simulink model "simulator_model_PVA_FINAL"  (R2016b)
settings: Solver=FixedStepAuto  StartTime=0.0  StopTime=t  FixedStep=0.005  RelTol=1e-3
StopFcn:
  | Plots
values from neighbouring files (symbols this model uses):
  a_cross = exp(-deltat/tau)    [simulation_script.m]
  a_long = a_cross    [simulation_script.m]
  a_vel_att = exp(-deltat/tau_vel_att)    [simulation_script.m]
  deltat = deltat_array(i)    [simulation_script.m]
  lat = latency(h)*0.001    [simulation_script.m]
  lat_acc = 3.25    [simulation_script.m]
  s_att = sqrt(1-a_vel_att^2)*s_att_e    [simulation_script.m]
  s_cross = sqrt(1-a_cross^2)*s_e(k)    [simulation_script.m]
  s_long = sqrt(1-a_long^2)*s_e1(k)    [simulation_script.m]
  s_vel = sqrt(1-a_vel_att^2)*s_vel_e    [simulation_script.m]
libraries: simulink x3
settings Model: Creator=trrrbe  LastModifiedBy=trrrbe
settings SolverCC: ZeroCrossAlgorithm=Adaptive
settings OptimizationCC: EfficientFloat2IntCast=on

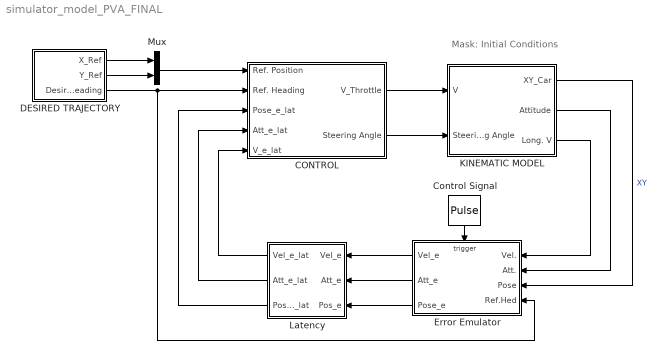
== system simulator_model_PVA_FINAL ==
  note: Mask: Initial Conditions
  CONTROL : Subsystem
  Control Signal : DiscretePulseGenerator  PulseType=Time based  Period=deltat  PulseWidth=50
  DESIRED TRAJECTORY : Subsystem  mask{n=3, A=100}
      mask prompts: n "Eccentricity"; A "Amplitude"
  Error Emulator : Subsystem
  KINEMATIC MODEL : Subsystem  mask{ref=0, x0=0, y0=0}
      mask prompts: ref "Reference Heading"; x0 "Initial Position X"; y0 "Initial Position Y"
  Latency : Subsystem
  Mux : Mux  Inputs=2
  wires:
  KINEMATIC MODEL/1(XY_Car) -> Error Emulator/3(Pose)  "XY"
  CONTROL/1(V_Throttle) -> KINEMATIC MODEL/1(V)
  DESIRED TRAJECTORY/1(X_Ref) -> Mux/1
  DESIRED TRAJECTORY/2(Y_Ref) -> Mux/2
  KINEMATIC MODEL/3(Long. V) -> Error Emulator/1(Vel.)
  KINEMATIC MODEL/2(Attitude) -> Error Emulator/2(Att.)
  DESIRED TRAJECTORY/3(Desired Heading) -> Error Emulator/4("Ref.Hed "), CONTROL/2(Ref. Heading)
  Control Signal/1 -> Error Emulator/Trigger
  Error Emulator/1(Vel_e) -> Latency/1(Vel_e)
  Error Emulator/3(Pose_e) -> Latency/3(Pos_e)
  CONTROL/2(Steering Angle) -> KINEMATIC MODEL/2(Steering Angle)
  Latency/3(Pos_e_lat) -> CONTROL/3(Pose_e_lat)
  Latency/1(Vel_e_lat) -> CONTROL/5(V_e_lat)
  Latency/2(Att_e_lat) -> CONTROL/4(Att_e_lat)
  Mux/1 -> CONTROL/1(Ref. Position)
  Error Emulator/2(Att_e) -> Latency/2(Att_e)

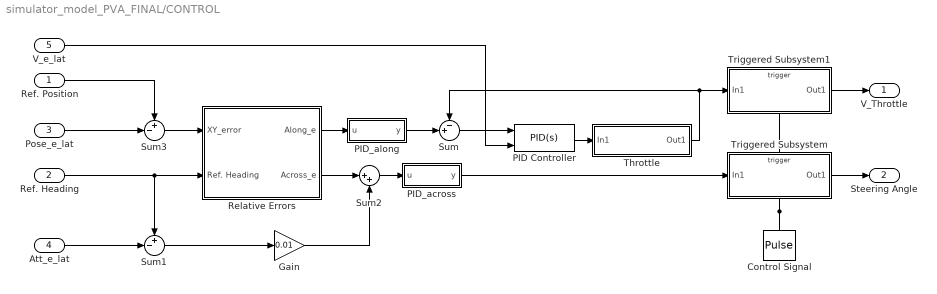
== system simulator_model_PVA_FINAL/CONTROL ==
  Ref. Position : Inport
  Ref. Heading : Inport  Port=2
  Pose_e_lat : Inport  Port=3
  Att_e_lat : Inport  Port=4
  V_e_lat : Inport  Port=5
  Control Signal : DiscretePulseGenerator  PulseType=Time based  Period=deltat  PulseWidth=50
  Gain : Gain  Gain=0.01
  PID Controller : simulink/Continuous/PID Controller  Controller=PID  TimeDomain=Continuous-time  SampleTime=-1  IntegratorMethod=Forward Euler  FilterMethod=Forward Euler  Form=Parallel  UseFilter=on  ControllerParametersSource=internal  P=209.609082036899  I=13.2325958582808  D=596.721506223276  N=1.87779602070702  InitialConditionSource=internal  InitialConditionForIntegrator=0  InitialConditionForFilter=0  ExternalReset=none  LimitOutput=off  UpperSaturationLimit=inf  LowerSaturationLimit=0  LinearizeAsGain=off  AntiWindupMode=clamping  Kb=1000  TrackingMode=on  Kt=t/500  PParamMin=[]  PParamMax=[]  IParamMin=[]  IParamMax=[]  DParamMin=[]  DParamMax=[]  NParamMin=[]  NParamMax=[]  KbParamMin=[]  KbParamMax=[]  KtParamMin=[]  KtParamMax=[]  POutMin=[]  POutMax=[]  IOutMin=[]  IOutMax=[]  DOutMin=[]  DOutMax=[]  NOutMin=[]  NOutMax=[]  KbOutMin=[]  KbOutMax=[]  KtOutMin=[]  KtOutMax=[]  IntegratorOutMin=[]  IntegratorOutMax=[]  FilterOutMin=[]  FilterOutMax=[]  SumOutMin=[]  SumOutMax=[]  SumI1OutMin=[]  SumI1OutMax=[]  SumI2OutMin=[]  SumI2OutMax=[]  SumI3OutMin=[]  SumI3OutMax=[]  SumDOutMin=[]  SumDOutMax=[]  SaturationOutMin=[]  SaturationOutMax=[]  IntegratorContinuousStateAttributes=''  IntegratorStateMustResolveToSignalObject=off  IntegratorRTWStateStorageClass=Auto  FilterContinuousStateAttributes=''  FilterStateMustResolveToSignalObject=off  FilterRTWStateStorageClass=Auto  DifferentiatorICPrevScaledInput=0  DifferentiatorOutMin=[]  DifferentiatorOutMax=[]
  PID_across : Subsystem
  PID_along : Subsystem
  Relative Errors : Subsystem
  Sum : Sum  Inputs=-+|
  Sum1 : Sum  Inputs=+-|
  Sum2 : Sum  Inputs=|++
  Sum3 : Sum  Inputs=+-|
  Throttle : Subsystem
  Triggered Subsystem : Subsystem  TreatAsAtomicUnit=on
  Triggered Subsystem1 : Subsystem  TreatAsAtomicUnit=on
  V_Throttle : Outport
  Steering Angle : Outport  Port=2
  wires:
  PID Controller/1 -> Throttle/1(In1)
  Sum/1 -> PID Controller/1
  Pose_e_lat/1 -> Sum3/2
  Ref. Position/1 -> Sum3/1
  Ref. Heading/1 -> Relative Errors/2(Ref. Heading), Sum1/1
  Att_e_lat/1 -> Sum1/2
  Throttle/1(Out1) -> Triggered Subsystem1/1(In1), Sum/1
  Triggered Subsystem/1(Out1) -> Steering Angle/1
  Control Signal/1 -> Triggered Subsystem/Trigger, Triggered Subsystem1/Trigger
  Sum3/1 -> Relative Errors/1(XY_error)
  Triggered Subsystem1/1(Out1) -> V_Throttle/1
  Relative Errors/1(Along_e) -> PID_along/1(u)
  Relative Errors/2(Across_e) -> Sum2/1
  PID_along/1(y) -> Sum/2
  Sum1/1 -> Gain/1
  V_e_lat/1 -> PID Controller/2
  Sum2/1 -> PID_across/1(u)
  PID_across/1(y) -> Triggered Subsystem/1(In1)
  Gain/1 -> Sum2/2

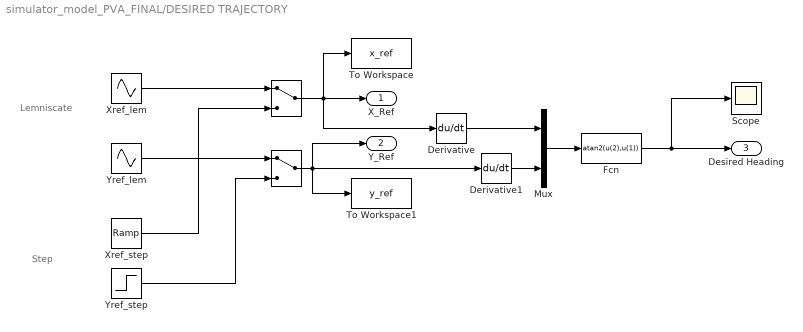
== system simulator_model_PVA_FINAL/DESIRED TRAJECTORY ==
  note: Step
  note: Lemniscate
  " " : ManualSwitch
  "  " : ManualSwitch
  Derivative : Derivative
  Derivative1 : Derivative
  Fcn : Fcn  Expr=atan2(u(2),u(1))
  Mux : Mux  Inputs=2
  Scope : Scope
  To Workspace : ToWorkspace  VariableName=x_ref  SaveFormat=Timeseries  SampleTime=-1
  To Workspace1 : ToWorkspace  VariableName=y_ref  SaveFormat=Timeseries  SampleTime=-1
  Xref_lem : Sin  Amplitude=n*A  Frequency=2*pi/t  SampleTime=0
  Xref_step : simulink/Sources/Ramp  slope=10  start=0  X0=0
  Yref_lem : Sin  Amplitude=A  Frequency=4*pi/t  SampleTime=0
  Yref_step : Step  Time=50  After=5  SampleTime=0
  X_Ref : Outport
  Y_Ref : Outport  Port=2
  Desired Heading : Outport  Port=3
  wires:
  Xref_lem/1 -> "  "/1
  Yref_lem/1 -> " "/1
  Xref_step/1 -> "  "/2
  " "/1 -> Y_Ref/1, To Workspace1/1, Derivative1/1
  Derivative/1 -> Mux/1
  Derivative1/1 -> Mux/2
  Mux/1 -> Fcn/1
  Fcn/1 -> Scope/1, Desired Heading/1
  "  "/1 -> To Workspace/1, X_Ref/1, Derivative/1
  Yref_step/1 -> " "/2

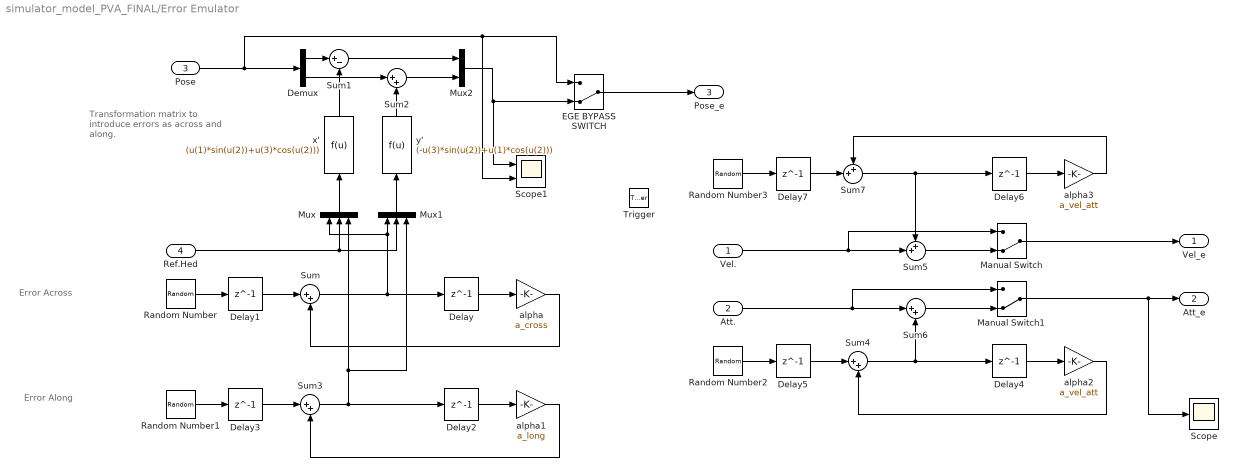
== system simulator_model_PVA_FINAL/Error Emulator ==
  note: Transformation matrix to
      | introduce errors as across
      | and along.
  note: Error Along
  note: Error Across
  Vel. : Inport
  Att. : Inport  Port=2
  Pose : Inport  Port=3
  "Ref.Hed " : Inport  Port=4
  Trigger : TriggerPort  VariantControl=Variant  PortDimensions=1
  Delay{,1..7} (8 alike) : Delay  DelayLength=1  InitialCondition=0
  Demux : Demux  Outputs=2
  EGE BYPASS SWITCH : ManualSwitch  CurrentSetting=0
  Manual Switch : ManualSwitch  CurrentSetting=0
  Manual Switch1 : ManualSwitch  CurrentSetting=0
  Mux : Mux  Inputs=3
  Mux1 : Mux  Inputs=3
  Mux2 : Mux  Inputs=2
  Random Number : RandomNumber  Variance=s_cross^2
  Random Number1 : RandomNumber  Variance=s_long^2
  Random Number2 : RandomNumber  Variance=s_att^2
  Random Number3 : RandomNumber  Variance=s_vel^2
  Scope : Scope
  Scope1 : Scope  NumInputPorts=2
  Sum{,2..4,6} (5 alike) : Sum  Inputs=|++
  Sum1 : Sum  Inputs=|+-
  Sum5 : Sum  Inputs=++|
  Sum7 : Sum  Inputs=++|
  alpha : Gain  Gain=a_cross
  alpha1 : Gain  Gain=a_long
  alpha2 : Gain  Gain=a_vel_att
  alpha3 : Gain  Gain=a_vel_att
  x' : Fcn  Expr=(u(1)*sin(u(2))+u(3)*cos(u(2)))
  y' : Fcn  Expr=(-u(3)*sin(u(2))+u(1)*cos(u(2)))
  Vel_e : Outport
  Att_e : Outport  Port=2
  Pose_e : Outport  Port=3
  wires:
  Random Number/1 -> Delay1/1
  Delay/1 -> alpha/1
  alpha/1 -> Sum/2
  Mux2/1 -> Scope1/1, EGE BYPASS SWITCH/2
  Mux1/1 -> y'/1
  Mux/1 -> x'/1
  "Ref.Hed "/1 -> Mux1/2, Mux/2
  Sum2/1 -> Mux2/2
  Sum1/1 -> Mux2/1
  x'/1 -> Sum1/2
  Demux/1 -> Sum1/1
  Demux/2 -> Sum2/1
  y'/1 -> Sum2/2
  Pose/1 -> Demux/1, Scope1/2, EGE BYPASS SWITCH/1
  Delay1/1 -> Sum/1
  Random Number1/1 -> Delay3/1
  Sum3/1 -> Delay2/1, Mux1/3, Mux/3
  Delay2/1 -> alpha1/1
  alpha1/1 -> Sum3/2
  Delay3/1 -> Sum3/1
  Sum/1 -> Mux1/1, Mux/1, Delay/1
  Random Number2/1 -> Delay5/1
  Sum4/1 -> Delay4/1, Sum6/2
  Delay4/1 -> alpha2/1
  alpha2/1 -> Sum4/2
  Delay5/1 -> Sum4/1
  Vel./1 -> Manual Switch/1, Sum5/2
  Att./1 -> Manual Switch1/1, Sum6/1
  Sum6/1 -> Manual Switch1/2
  alpha3/1 -> Sum7/1
  Sum7/1 -> Delay6/1, Sum5/1
  Random Number3/1 -> Delay7/1
  Delay7/1 -> Sum7/2
  Delay6/1 -> alpha3/1
  Sum5/1 -> Manual Switch/2
  EGE BYPASS SWITCH/1 -> Pose_e/1
  Manual Switch/1 -> Vel_e/1
  Manual Switch1/1 -> Scope/1, Att_e/1

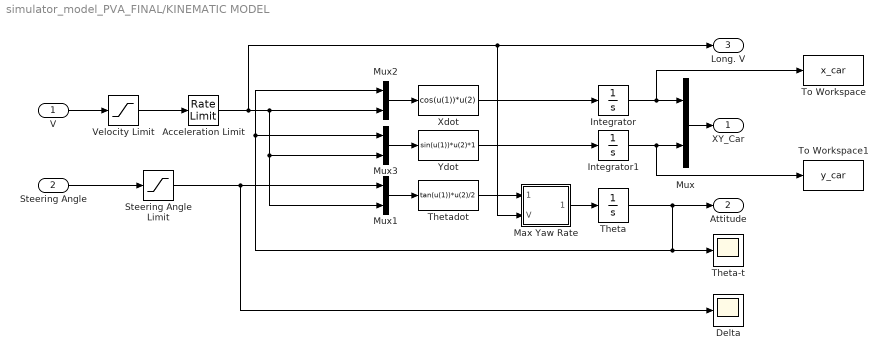
== system simulator_model_PVA_FINAL/KINEMATIC MODEL ==
  V : Inport
  Steering Angle : Inport  Port=2
  Acceleration Limit : RateLimiter  RisingSlewLimit=3  FallingSlewLimit=-3  SampleTimeMode=inherited
  Delta : Scope
  Integrator : Integrator  InitialCondition=x0
  Integrator1 : Integrator  InitialCondition=y0
  Max Yaw Rate : Subsystem
  Mux{,1..3} (4 alike) : Mux  Inputs=2
  Steering Angle Limit : Saturate  UpperLimit=pi/4  LowerLimit=-pi/4
  Theta : Integrator  InitialCondition=ref
  Theta-t : Scope
  Thetadot : Fcn  Expr=tan(u(1))*u(2)/2
  To Workspace : ToWorkspace  VariableName=x_car  SaveFormat=Timeseries  SampleTime=-1
  To Workspace1 : ToWorkspace  VariableName=y_car  SaveFormat=Timeseries  SampleTime=-1
  Velocity Limit : Saturate  UpperLimit=25  LowerLimit=0
  Xdot : Fcn  Expr=cos(u(1))*u(2)
  Ydot : Fcn  Expr=sin(u(1))*u(2)*1
  XY_Car : Outport
  Attitude : Outport  Port=2
  Long. V : Outport  Port=3
  wires:
  Thetadot/1 -> Max Yaw Rate/1(theta_dot)
  Xdot/1 -> Integrator/1
  Mux1/1 -> Thetadot/1
  Mux2/1 -> Xdot/1
  Mux3/1 -> Ydot/1
  Mux/1 -> XY_Car/1
  Integrator1/1 -> To Workspace1/1, Mux/2
  Integrator/1 -> Mux/1, To Workspace/1
  Ydot/1 -> Integrator1/1
  V/1 -> Velocity Limit/1
  Velocity Limit/1 -> Acceleration Limit/1
  Steering Angle/1 -> Steering Angle Limit/1
  Theta/1 -> Attitude/1, Mux3/1, Mux2/1, Theta-t/1
  Max Yaw Rate/1(theta_dot_sat) -> Theta/1
  Steering Angle Limit/1 -> Delta/1, Mux1/1
  Acceleration Limit/1 -> Max Yaw Rate/2(V), Long. V/1, Mux2/2, Mux1/2, Mux3/2

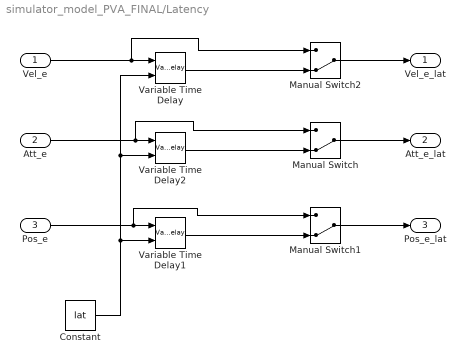
== system simulator_model_PVA_FINAL/Latency ==
  Vel_e : Inport
  Att_e : Inport  Port=2
  Pos_e : Inport  Port=3
  Constant : Constant  Value=lat
  Manual Switch : ManualSwitch  CurrentSetting=0
  Manual Switch1 : ManualSwitch  CurrentSetting=0
  Manual Switch2 : ManualSwitch  CurrentSetting=0
  Variable Time Delay : VariableTransportDelay  MaximumDelay=20  ZeroDelay=on
  Variable Time Delay1 : VariableTransportDelay  MaximumDelay=20  ZeroDelay=on
  Variable Time Delay2 : VariableTransportDelay  MaximumDelay=20  ZeroDelay=on
  Vel_e_lat : Outport
  Att_e_lat : Outport  Port=2
  Pos_e_lat : Outport  Port=3
  wires:
  Vel_e/1 -> Manual Switch2/1, Variable Time Delay/1
  Att_e/1 -> Manual Switch/1, Variable Time Delay2/1
  Pos_e/1 -> Manual Switch1/1, Variable Time Delay1/1
  Variable Time Delay2/1 -> Manual Switch/2
  Variable Time Delay1/1 -> Manual Switch1/2
  Variable Time Delay/1 -> Manual Switch2/2
  Constant/1 -> Variable Time Delay1/2, Variable Time Delay2/2, Variable Time Delay/2
  Manual Switch2/1 -> Vel_e_lat/1
  Manual Switch/1 -> Att_e_lat/1
  Manual Switch1/1 -> Pos_e_lat/1

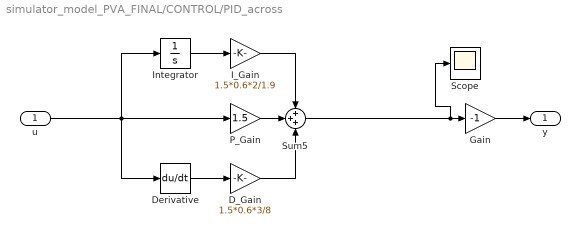
== system simulator_model_PVA_FINAL/CONTROL/PID_across ==
  u : Inport
  D_Gain : Gain  Gain=1.5*0.6*3/8
  Derivative : Derivative
  Gain : Gain  Gain=-1
  I_Gain : Gain  Gain=1.5*0.6*2/1.9
  Integrator : Integrator  WrapState=on  WrappedStateUpperValue=pi/10  WrappedStateLowerValue=-pi/10
  P_Gain : Gain  Gain=1.5
  Scope : Scope
  Sum5 : Sum  Inputs=+++
  y : Outport
  wires:
  P_Gain/1 -> Sum5/2
  Derivative/1 -> D_Gain/1
  D_Gain/1 -> Sum5/3
  Integrator/1 -> I_Gain/1
  I_Gain/1 -> Sum5/1
  u/1 -> P_Gain/1, Integrator/1, Derivative/1
  Sum5/1 -> Scope/1, Gain/1
  Gain/1 -> y/1

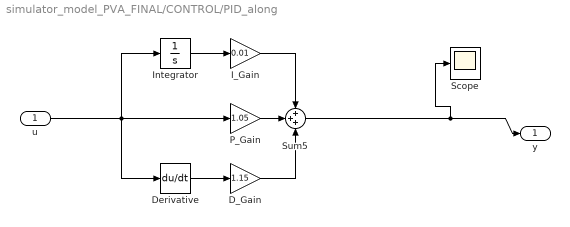
== system simulator_model_PVA_FINAL/CONTROL/PID_along ==
  u : Inport
  D_Gain : Gain  Gain=1.15
  Derivative : Derivative
  I_Gain : Gain  Gain=0.01
  Integrator : Integrator
  P_Gain : Gain  Gain=1.05
  Scope : Scope
  Sum5 : Sum  Inputs=+++
  y : Outport
  wires:
  P_Gain/1 -> Sum5/2
  Derivative/1 -> D_Gain/1
  D_Gain/1 -> Sum5/3
  Integrator/1 -> I_Gain/1
  I_Gain/1 -> Sum5/1
  u/1 -> P_Gain/1, Integrator/1, Derivative/1
  Sum5/1 -> Scope/1, y/1

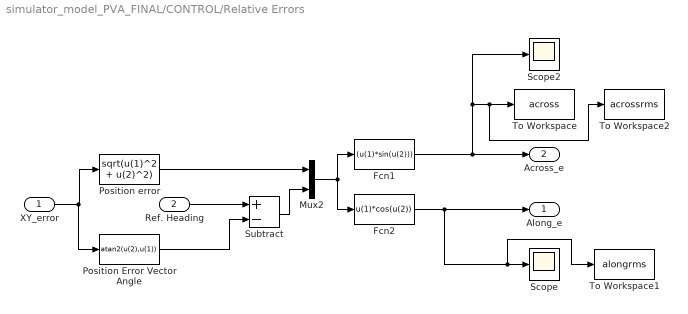
== system simulator_model_PVA_FINAL/CONTROL/Relative Errors ==
  XY_error : Inport
  Ref. Heading : Inport  Port=2
  Fcn1 : Fcn  Expr=(u(1)*sin(u(2)))
  Fcn2 : Fcn  Expr=u(1)*cos(u(2))
  Mux2 : Mux  Inputs=2
  Position Error Vector Angle : Fcn  Expr=atan2(u(2),u(1))
  Position error : Fcn  Expr=sqrt(u(1)^2 + u(2)^2)
  Scope : Scope
  Scope2 : Scope
  Subtract : Sum  Inputs=+-
  To Workspace : ToWorkspace  VariableName=across  SaveFormat=Timeseries  SampleTime=-1
  To Workspace1 : ToWorkspace  VariableName=alongrms  SampleTime=-1
      settings: Save2DSignal=2-D array (concatenate along first dimension)
  To Workspace2 : ToWorkspace  VariableName=acrossrms  SampleTime=-1
      settings: Save2DSignal=2-D array (concatenate along first dimension)
  Along_e : Outport
  Across_e : Outport  Port=2
  wires:
  Position error/1 -> Mux2/1
  Position Error Vector Angle/1 -> Subtract/2
  Subtract/1 -> Mux2/2
  Mux2/1 -> Fcn2/1, Fcn1/1
  Ref. Heading/1 -> Subtract/1
  XY_error/1 -> Position Error Vector Angle/1, Position error/1
  Fcn1/1 -> Across_e/1, Scope2/1, To Workspace2/1, To Workspace/1
  Fcn2/1 -> To Workspace1/1, Scope/1, Along_e/1

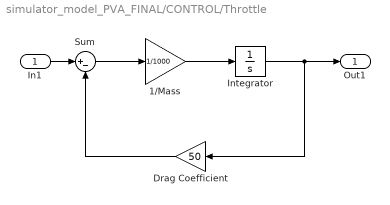
== system simulator_model_PVA_FINAL/CONTROL/Throttle ==
  In1 : Inport
  1/Mass : Gain  Gain=1/1000
  Drag Coefficient : Gain  Gain=50
  Integrator : Integrator  InitialCondition=5
  Sum : Sum  Inputs=|+-
  Out1 : Outport
  wires:
  1/Mass/1 -> Integrator/1
  Integrator/1 -> Out1/1, Drag Coefficient/1
  In1/1 -> Sum/1
  Drag Coefficient/1 -> Sum/2
  Sum/1 -> 1/Mass/1

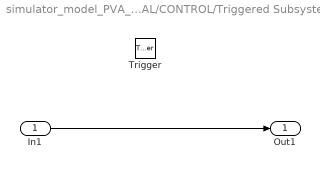
== system simulator_model_PVA_FINAL/CONTROL/Triggered Subsystem ==
  In1 : Inport
  Trigger : TriggerPort  VariantControl=Variant
  Out1 : Outport
  wires:
  In1/1 -> Out1/1

== system simulator_model_PVA_FINAL/CONTROL/Triggered Subsystem1 ==
  In1 : Inport
  Trigger : TriggerPort  VariantControl=Variant
  Out1 : Outport
  wires:
  In1/1 -> Out1/1

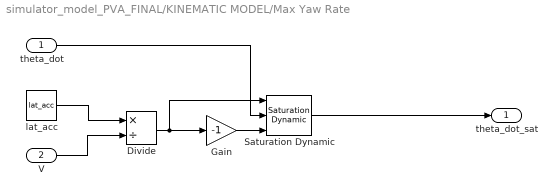
== system simulator_model_PVA_FINAL/KINEMATIC MODEL/Max Yaw Rate ==
  theta_dot : Inport
  V : Inport  Port=2
  Divide : Product  Inputs=*/
  Gain : Gain  Gain=-1
  Saturation Dynamic : simulink/Discontinuities/Saturation Dynamic  OutMin=[]  OutMax=[]  OutDataTypeStr=Inherit: Same as second input  OutDataType=fixdt(1, 16)  OutScaling=2^-10  DoSatur=off
  lat_acc : Constant  Value=lat_acc
  theta_dot_sat : Outport
  wires:
  theta_dot/1 -> Saturation Dynamic/2
  V/1 -> Divide/2
  lat_acc/1 -> Divide/1
  Divide/1 -> Gain/1, Saturation Dynamic/1
  Gain/1 -> Saturation Dynamic/3
  Saturation Dynamic/1 -> theta_dot_sat/1
